simulink model "sample1_cw_acw2_signal"  (R2021b)
settings: Solver=FixedStepDiscrete  StartTime=0.0  StopTime=255*2  FixedStep=1  RelTol=1e-3
libraries: simulink x1
settings Model: Creator=kawata  LastModifiedBy=kawata
settings DataIOCC: ReturnWorkspaceOutputs=off

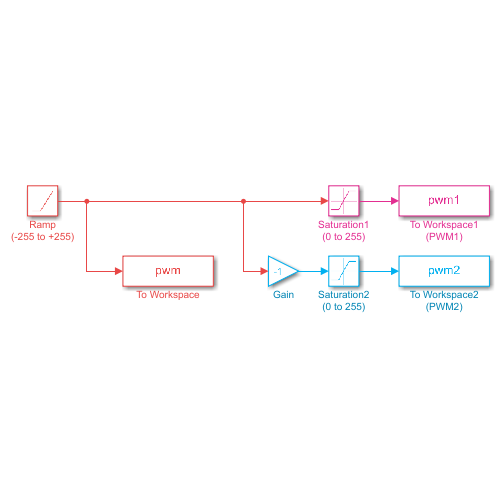
[thumbnail: Simulink's stored preview of the top-level diagram]
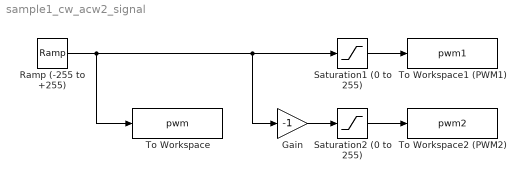
== system sample1_cw_acw2_signal ==
  Gain : Gain  Gain=-1
  Ramp (-255 to +255) : simulink/Sources/Ramp  slope=1  start=0  InitialOutput=-255
  Saturation1 (0 to 255) : Saturate  UpperLimit=255  LowerLimit=0
  Saturation2 (0 to 255) : Saturate  UpperLimit=255  LowerLimit=0
  To Workspace : ToWorkspace  VariableName=pwm  SampleTime=-1
  To Workspace1 (PWM1) : ToWorkspace  VariableName=pwm1  SampleTime=-1
  To Workspace2 (PWM2) : ToWorkspace  VariableName=pwm2  SampleTime=-1
  wires:
  Ramp (-255 to +255)/1 -> To Workspace/1, Saturation1 (0 to 255)/1, Gain/1
  Saturation1 (0 to 255)/1 -> To Workspace1 (PWM1)/1
  Saturation2 (0 to 255)/1 -> To Workspace2 (PWM2)/1
  Gain/1 -> Saturation2 (0 to 255)/1
